simulink model "steuerung"  (R2016b)
settings: Solver=VariableStepAuto  StartTime=0.0  StopTime=inf  RelTol=1e-3
settings Model: Creator=Patrick  LastModifiedBy=Patrick

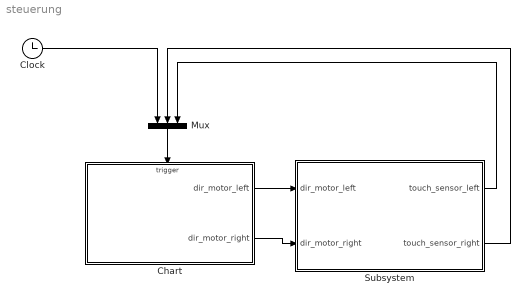
== system steuerung ==
  Chart : Stateflow chart  TreatAsAtomicUnit=on
  Clock : Clock
  Mux : Mux  Inputs=3
  Subsystem : Subsystem
  wires:
  Clock/1 -> Mux/1
  Mux/1 -> Chart/Trigger
  Chart/1(dir_motor_left) -> Subsystem/1(dir_motor_left)
  Chart/2(dir_motor_right) -> Subsystem/2(dir_motor_right)
  Subsystem/1(touch_sensor_left) -> Mux/3
  Subsystem/2(touch_sensor_right) -> Mux/2

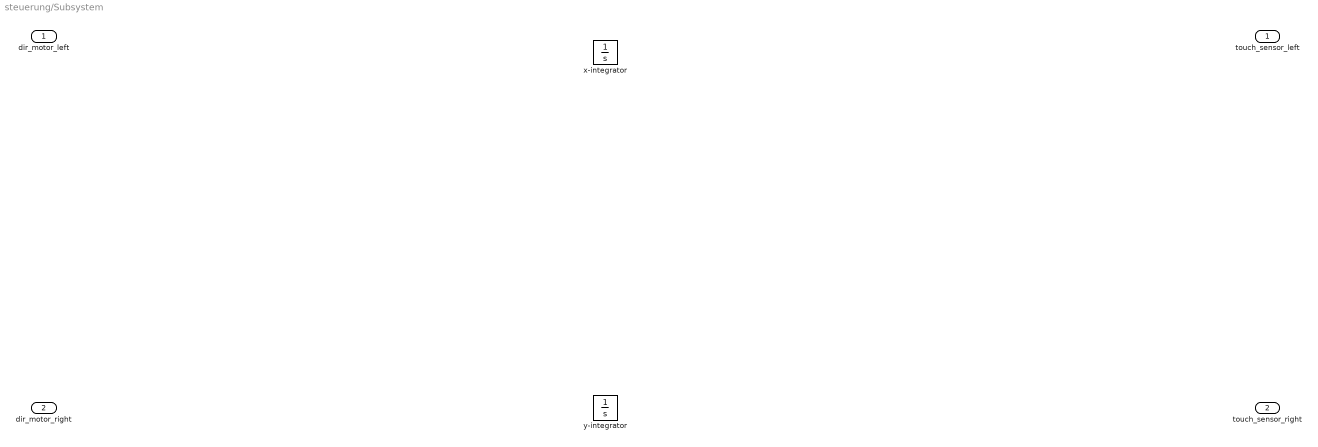
== system steuerung/Subsystem ==
  dir_motor_left : Inport
  dir_motor_right : Inport  Port=2
  x-integrator : Integrator
  y-integrator : Integrator
  touch_sensor_left : Outport
  touch_sensor_right : Outport  Port=2

== stateflow chart steuerung/Chart ==
  state FORWARD
    entry:
    dir_motor_left=1;
    dir_motor_right=1;
  state TURN_LEFT
    entry:
    dir_motor_left=2;
    dir_motor_right=1;
  state TURN_RIGHT
    entry:
    dir_motor_left=1;
    dir_motor_right=2;
  state BACKWARD
    entry:
    dir_motor_left=2;
    dir_motor_right=2;
    state LEFT
    state RIGHT
    (default) -> RIGHT
  (default) -> FORWARD
  TURN_LEFT -> FORWARD : after(T_TURN, SysClock)
  TURN_RIGHT -> FORWARD : after(T_TURN, SysClock)
  FORWARD -> LEFT [order 1] : touch_sensor_right
  FORWARD -> RIGHT [order 2] : touch_sensor_left
  LEFT -> TURN_LEFT : after(T_BACK, SysClock)
  RIGHT -> TURN_RIGHT : after(T_BACK,SysClock)
  data: dir_motor_left output; dir_motor_right output
  events: touch_sensor_left input RISING_EDGE_EVENT; touch_sensor_right input RISING_EDGE_EVENT
